simulink model "point_mass_subsonic_airplane"  (R2024b)
settings: Solver=ode45  StartTime=0.0  StopTime=5*60  RelTol=1e-6  AbsTol=1e-9
values from neighbouring files (symbols this model uses):
  FPS2MPH = 3600/5280    (= 0.681818181818)    [luckep2.m]
  RAD2DEG = 180/pi    (= 57.2957795131)    [luckep2.m]
undefined symbols (not defined in the file or in its folder): gd, ic, params
libraries: simulink_extras x5, dspstat3 x1, simulink x1
settings Model: Creator=jdlarson1  LastModifiedBy=Benjamin Lucke
settings SolverCC: AlgebraicLoopSolver=TrustRegion
settings DataIOCC: SaveFormat=Array  SignalLoggingSaveFormat=ModelDataLogs  ReturnWorkspaceOutputs=off
settings OptimizationCC: BlockReduction=off  BooleanDataType=off  ReuseModelBlockBuffer=off
settings DebuggingCC: SaveWithParameterizedLinksMsg=none  UnderspecifiedInitializationDetection=Classic  MergeDetectMultiDrivingBlocksExec=none  SignalResolutionControl=TryResolveAllWithWarning  MultiTaskDSMMsg=warning  MultiTaskCondExecSysMsg=none  UnconnectedInputMsg=warning  UnconnectedOutputMsg=warning  UnconnectedLineMsg=warning
settings HardwareCC: TargetUnknown=on
settings ModelReferenceCC: EnableRefExpFcnMdlSchedulingChecks=on  PropagateSignalLabelsOutOfModel=off
settings RTWCC: GPUComputeCapability=3.5  DLArmComputeVersion=19.05
settings GRTTargetCC: CombineOutputUpdateFcns=off  GRTInterface=on

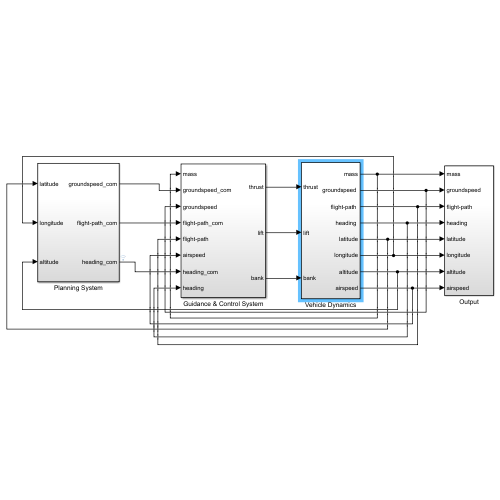
[thumbnail: Simulink's stored preview of the top-level diagram]
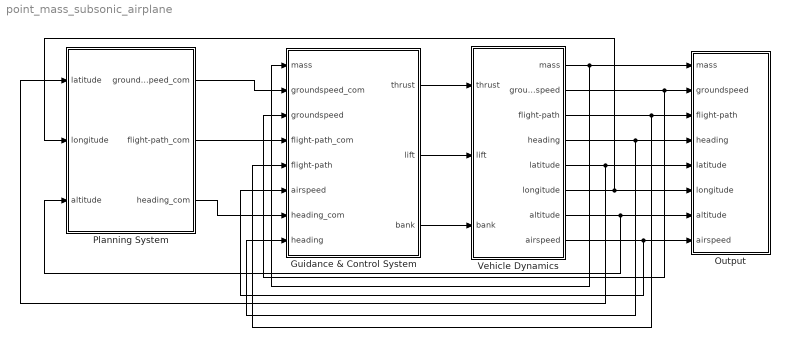
== system point_mass_subsonic_airplane ==
  Guidance & Control System : Subsystem
  Output : Subsystem
  Planning System : Subsystem
  Vehicle Dynamics : Subsystem
  wires:
  Guidance & Control System/3(bank) -> Vehicle Dynamics/3(bank)
  Vehicle Dynamics/1(" mass") -> Output/1(mass), Guidance & Control System/1(mass)
  Guidance & Control System/2(lift) -> Vehicle Dynamics/2("lift ")
  Guidance & Control System/1(thrust) -> Vehicle Dynamics/1("thrust ")
  Planning System/1(groundspeed_com) -> Guidance & Control System/2(groundspeed_com)
  Planning System/2(flight-path_com) -> Guidance & Control System/4(flight-path_com)
  Planning System/3(heading_com) -> Guidance & Control System/7(heading_com)
  Vehicle Dynamics/4(" heading ") -> Guidance & Control System/8(heading), Output/4(heading)
  Vehicle Dynamics/3(" flight-path ") -> Guidance & Control System/5(flight-path), Output/3(flight-path)
  Vehicle Dynamics/2(" groundspeed ") -> Guidance & Control System/3(groundspeed), Output/2(groundspeed)
  Vehicle Dynamics/8(airspeed) -> Guidance & Control System/6(airspeed), Output/8(airspeed)
  Vehicle Dynamics/7(altitude) -> Planning System/3(altitude), Output/7(altitude)
  Vehicle Dynamics/6(longitude) -> Planning System/2(longitude), Output/6(longitude)
  Vehicle Dynamics/5(latitude) -> Planning System/1(latitude), Output/5(latitude)

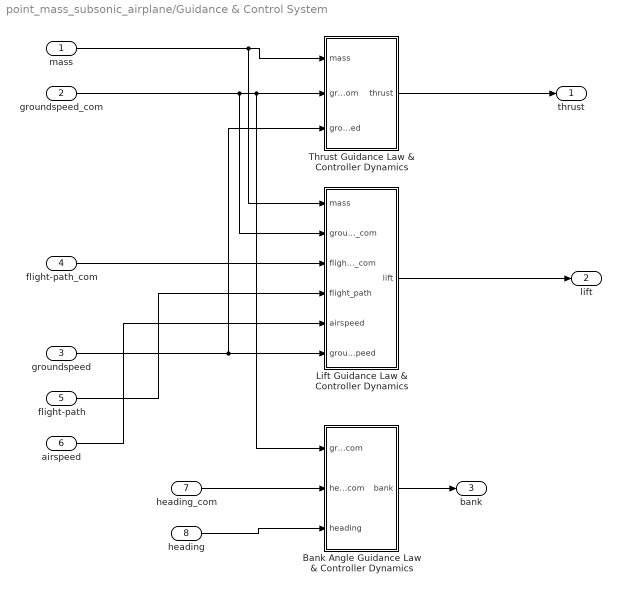
== system point_mass_subsonic_airplane/Guidance & Control System ==
  mass : Inport
  groundspeed_com : Inport  Port=2
  groundspeed : Inport  Port=3
  flight-path_com : Inport  Port=4
  flight-path : Inport  Port=5
  airspeed : Inport  Port=6
  heading_com : Inport  Port=7
  heading : Inport  Port=8
  Bank Angle Guidance Law & Controller Dynamics : Subsystem
  Lift Guidance Law & Controller Dynamics : Subsystem
  Thrust Guidance Law & Controller Dynamics : Subsystem
  thrust : Outport
  lift : Outport  Port=2
  bank : Outport  Port=3
  wires:
  mass/1 -> Lift Guidance Law & Controller Dynamics/1(mass), Thrust Guidance Law & Controller Dynamics/1(mass)
  flight-path_com/1 -> Lift Guidance Law & Controller Dynamics/3(flight_path_com)
  flight-path/1 -> Lift Guidance Law & Controller Dynamics/4(flight_path)
  groundspeed/1 -> Thrust Guidance Law & Controller Dynamics/3(groundspeed), Lift Guidance Law & Controller Dynamics/6(groundspeed)
  groundspeed_com/1 -> Bank Angle Guidance Law & Controller Dynamics/1(groundspeed_com), Thrust Guidance Law & Controller Dynamics/2(groundspeed_com), Lift Guidance Law & Controller Dynamics/2(groundspeed_com)
  heading/1 -> Bank Angle Guidance Law & Controller Dynamics/3(heading)
  airspeed/1 -> Lift Guidance Law & Controller Dynamics/5(airspeed)
  heading_com/1 -> Bank Angle Guidance Law & Controller Dynamics/2(heading_com)
  Thrust Guidance Law & Controller Dynamics/1(thrust) -> thrust/1
  Lift Guidance Law & Controller Dynamics/1(lift) -> lift/1
  Bank Angle Guidance Law & Controller Dynamics/1(bank) -> bank/1

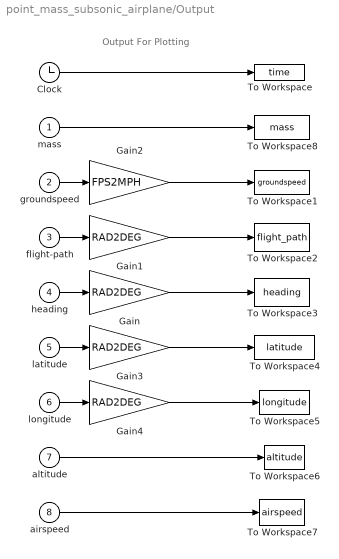
== system point_mass_subsonic_airplane/Output ==
  note: Output For Plotting
  mass : Inport
  groundspeed : Inport  Port=2
  flight-path : Inport  Port=3
  heading : Inport  Port=4
  latitude : Inport  Port=5
  longitude : Inport  Port=6
  altitude : Inport  Port=7
  airspeed : Inport  Port=8
  Clock : Clock
  Gain{,1,3..4} (4 alike) : Gain  Gain=RAD2DEG
  Gain2 : Gain  Gain=FPS2MPH
  To Workspace : ToWorkspace  VariableName=time
  To Workspace1 : ToWorkspace  VariableName=groundspeed
  To Workspace2 : ToWorkspace  VariableName=flight_path
  To Workspace3 : ToWorkspace  VariableName=heading
  To Workspace4 : ToWorkspace  VariableName=latitude
  To Workspace5 : ToWorkspace  VariableName=longitude
  To Workspace6 : ToWorkspace  VariableName=altitude
  To Workspace7 : ToWorkspace  VariableName=airspeed
  To Workspace8 : ToWorkspace  VariableName=mass
  wires:
  Clock/1 -> To Workspace/1
  latitude/1 -> Gain3/1
  groundspeed/1 -> Gain2/1
  flight-path/1 -> Gain1/1
  heading/1 -> Gain/1
  longitude/1 -> Gain4/1
  altitude/1 -> To Workspace6/1
  Gain2/1 -> To Workspace1/1
  Gain1/1 -> To Workspace2/1
  Gain/1 -> To Workspace3/1
  airspeed/1 -> To Workspace7/1
  mass/1 -> To Workspace8/1
  Gain3/1 -> To Workspace4/1
  Gain4/1 -> To Workspace5/1

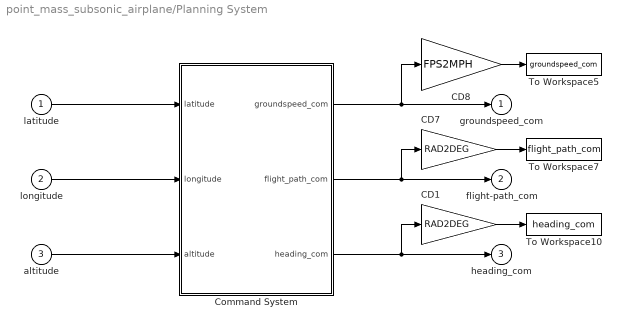
== system point_mass_subsonic_airplane/Planning System ==
  latitude : Inport
  longitude : Inport  Port=2
  altitude : Inport  Port=3
  CD1 : Gain  Gain=RAD2DEG  SaturateOnIntegerOverflow=on
  CD7 : Gain  Gain=RAD2DEG  SaturateOnIntegerOverflow=on
  CD8 : Gain  Gain=FPS2MPH  SaturateOnIntegerOverflow=on
  Command System : MATLAB Function  TreatAsAtomicUnit=on
  To Workspace10 : ToWorkspace  VariableName=heading_com
  To Workspace5 : ToWorkspace  VariableName=groundspeed_com
  To Workspace7 : ToWorkspace  VariableName=flight_path_com
  groundspeed_com : Outport
  flight-path_com : Outport  Port=2
  heading_com : Outport  Port=3
  wires:
  longitude/1 -> Command System/2(longitude)
  altitude/1 -> Command System/3(altitude)
  Command System/1(groundspeed_com) -> CD8/1, groundspeed_com/1
  Command System/2(flight_path_com) -> CD7/1, flight-path_com/1
  Command System/3(heading_com) -> CD1/1, heading_com/1
  CD8/1 -> To Workspace5/1
  CD7/1 -> To Workspace7/1
  CD1/1 -> To Workspace10/1
  latitude/1 -> Command System/1(latitude)

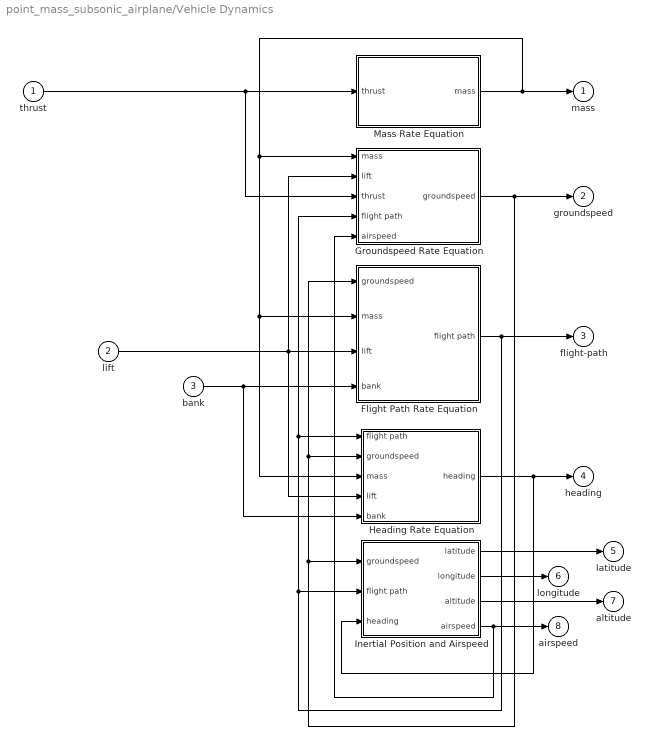
== system point_mass_subsonic_airplane/Vehicle Dynamics ==
  "thrust " : Inport
  "lift " : Inport  Port=2
  bank : Inport  Port=3
  Flight Path Rate Equation : Subsystem
  Groundspeed Rate Equation : Subsystem
  Heading Rate Equation : Subsystem
  Inertial Position and Airspeed : Subsystem
  Mass Rate Equation : Subsystem
  " mass" : Outport
  " groundspeed " : Outport  Port=2
  " flight-path " : Outport  Port=3
  " heading " : Outport  Port=4
  latitude : Outport  Port=5
  longitude : Outport  Port=6
  altitude : Outport  Port=7
  airspeed : Outport  Port=8
  wires:
  bank/1 -> Heading Rate Equation/5(bank), Flight Path Rate Equation/4(bank)
  "lift "/1 -> Heading Rate Equation/4("lift "), Flight Path Rate Equation/3("lift "), Groundspeed Rate Equation/2(lift)
  "thrust "/1 -> Groundspeed Rate Equation/3(thrust), Mass Rate Equation/1(thrust)
  Heading Rate Equation/1(heading) -> Inertial Position and Airspeed/3(heading), " heading "/1
  Flight Path Rate Equation/1(flight path) -> Groundspeed Rate Equation/4(flight path), Heading Rate Equation/1(flight path), Inertial Position and Airspeed/2("flight path "), " flight-path "/1
  Groundspeed Rate Equation/1(groundspeed) -> Flight Path Rate Equation/1(groundspeed), Heading Rate Equation/2(groundspeed), Inertial Position and Airspeed/1(groundspeed), " groundspeed "/1
  Inertial Position and Airspeed/2(longitude) -> longitude/1
  Inertial Position and Airspeed/4(airspeed) -> Groundspeed Rate Equation/5(airspeed), airspeed/1
  Inertial Position and Airspeed/1(latitude) -> latitude/1
  Inertial Position and Airspeed/3(altitude) -> altitude/1
  Mass Rate Equation/1("mass ") -> Heading Rate Equation/3(mass), Flight Path Rate Equation/2(mass), Groundspeed Rate Equation/1(mass), " mass"/1

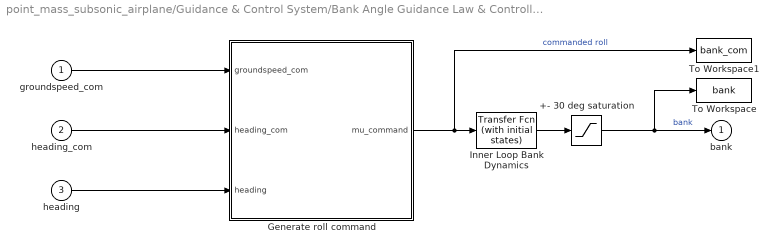
== system point_mass_subsonic_airplane/Guidance & Control System/Bank Angle Guidance Law & Controller Dynamics ==
  groundspeed_com : Inport
  heading_com : Inport  Port=2
  heading : Inport  Port=3
  +- 30 deg saturation : Saturate  UpperLimit=30*pi/180  LowerLimit=-30*pi/180
  Generate roll command : Subsystem
  Inner Loop Bank Dynamics : simulink_extras/Additional Linear/Transfer Fcn (with initial states)  N=[params.wu]  D="[1  params.wu]"  X0=0
  To Workspace : ToWorkspace  VariableName=bank
  To Workspace1 : ToWorkspace  VariableName=bank_com
  bank : Outport
  wires:
  groundspeed_com/1 -> Generate roll command/1(groundspeed_com)
  heading_com/1 -> Generate roll command/2(heading_com)
  heading/1 -> Generate roll command/3(heading)
  Generate roll command/1(mu_command) -> To Workspace1/1, Inner Loop Bank Dynamics/1  "commanded roll"
  Inner Loop Bank Dynamics/1 -> +- 30 deg saturation/1
  +- 30 deg saturation/1 -> bank/1, To Workspace/1  "bank"

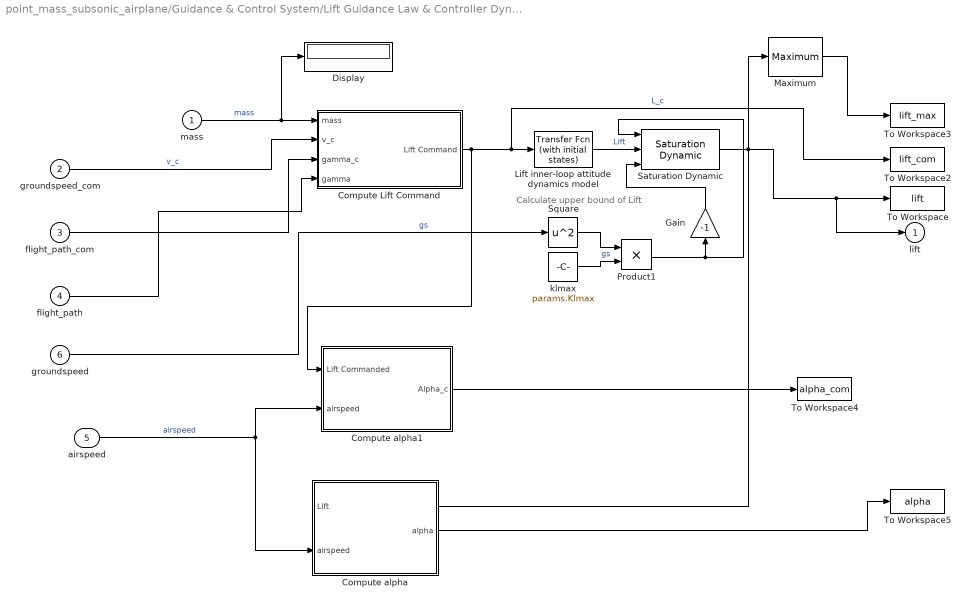
== system point_mass_subsonic_airplane/Guidance & Control System/Lift Guidance Law & Controller Dynamics ==
  note: Calculate upper bound of Lift
  mass : Inport
  groundspeed_com : Inport  Port=2
  flight_path_com : Inport  Port=3
  flight_path : Inport  Port=4
  airspeed : Inport  Port=5
  groundspeed : Inport  Port=6
  Compute Lift Command : Subsystem
  Compute alpha : Subsystem
  Compute alpha1 : Subsystem
  Display : Display
  Gain : Gain  Gain=-1
  Lift inner-loop attitude dynamics model : simulink_extras/Additional Linear/Transfer Fcn (with initial states)  N=[params.wl]  D="[1  params.wl]"  X0=0
  Maximum : dspstat3/Maximum  operation=maximum  fcn=Value  indexBase=One  operateOver=Each column  Dimension=1  InputProcessing=Columns as channels (frame based)  reset=None  roiEnable=off  roiType=Rectangles  roiPortion=Entire ROI  roiOutput=Individual statistics for each ROI  roiFlag=off  roundingMode=Floor  overflowMode=off  accumDataTypeStr=Inherit: Same as product output  accumLastDataTypeStr=Inherit: Same as product output
      settings: LibrarySourceBlock=dsphdlsupportstat/Maximum
  Product1 : Product
  Saturation Dynamic : simulink/Discontinuities/Saturation Dynamic  OutMin=[]  OutMax=[]  OutDataTypeStr=Inherit: Same as second input  OutDataType=fixdt(1, 16)  OutScaling=2^-10  DoSatur=off
  Square : Math  Operator=square
  To Workspace : ToWorkspace  VariableName=lift
  To Workspace2 : ToWorkspace  VariableName=lift_com
  To Workspace3 : ToWorkspace  VariableName=lift_max
  To Workspace4 : ToWorkspace  VariableName=alpha_com
  To Workspace5 : ToWorkspace  VariableName=alpha
  klmax : Constant  Value=params.Klmax
  lift : Outport
  wires:
  mass/1 -> Display/1, Compute Lift Command/1(mass)  "mass"
  groundspeed_com/1 -> Compute Lift Command/2(v_c)  "v_c"
  flight_path_com/1 -> Compute Lift Command/3(gamma_c)
  flight_path/1 -> Compute Lift Command/4(gamma)
  Compute Lift Command/1(Lift Command) -> Compute alpha1/1(Lift Commanded), To Workspace2/1, Lift inner-loop attitude dynamics model/1  "L_c"
  Lift inner-loop attitude dynamics model/1 -> Saturation Dynamic/2  "Lift"
  Maximum/1 -> To Workspace3/1
  groundspeed/1 -> Square/1  "gs"
  Square/1 -> Product1/1  "gs"
  klmax/1 -> Product1/2
  Product1/1 -> Gain/1, Saturation Dynamic/1
  Saturation Dynamic/1 -> Compute alpha/1(Lift), lift/1, To Workspace/1, Maximum/1
  airspeed/1 -> Compute alpha1/2(airspeed), Compute alpha/2(airspeed)  "airspeed"
  Compute alpha1/1(Alpha_c) -> To Workspace4/1
  Compute alpha/1(alpha) -> To Workspace5/1
  Gain/1 -> Saturation Dynamic/3

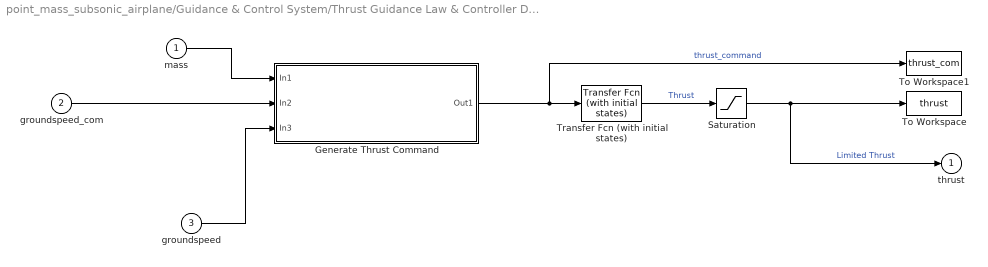
== system point_mass_subsonic_airplane/Guidance & Control System/Thrust Guidance Law & Controller Dynamics ==
  mass : Inport
  groundspeed_com : Inport  Port=2
  groundspeed : Inport  Port=3
  Generate Thrust Command : Subsystem
  Saturation : Saturate  UpperLimit=params.Tmax  LowerLimit=0
  To Workspace : ToWorkspace  VariableName=thrust
  To Workspace1 : ToWorkspace  VariableName=thrust_com
  Transfer Fcn (with initial states) : simulink_extras/Additional Linear/Transfer Fcn (with initial states)  N=[params.wt]  D="[1  params.wt]"  X0=22000
  thrust : Outport
  wires:
  mass/1 -> Generate Thrust Command/1(In1)
  groundspeed_com/1 -> Generate Thrust Command/2(In2)
  groundspeed/1 -> Generate Thrust Command/3(In3)
  Generate Thrust Command/1(Out1) -> Transfer Fcn (with initial states)/1, To Workspace1/1  "thrust_command"
  Transfer Fcn (with initial states)/1 -> Saturation/1  "Thrust"
  Saturation/1 -> thrust/1, To Workspace/1  "Limited Thrust"

== system point_mass_subsonic_airplane/Vehicle Dynamics/Flight Path Rate Equation ==
  groundspeed : Inport
  mass : Inport  Port=2
  "lift " : Inport  Port=3
  bank : Inport  Port=4
  Constant : Constant  Value=ic.g0
  Integrator : Integrator  InitialCondition=.05
  MATLAB Function : MATLAB Function  TreatAsAtomicUnit=on
  flight path : Outport
  wires:
  groundspeed/1 -> MATLAB Function/1(groundspeed)
  mass/1 -> MATLAB Function/2(mass)
  "lift "/1 -> MATLAB Function/3(lift)
  bank/1 -> MATLAB Function/4(bank)
  Constant/1 -> MATLAB Function/6(g0)
  MATLAB Function/1(flight_path_out) -> Integrator/1  "gamma_dot"
  Integrator/1 -> MATLAB Function/5(gamma), flight path/1

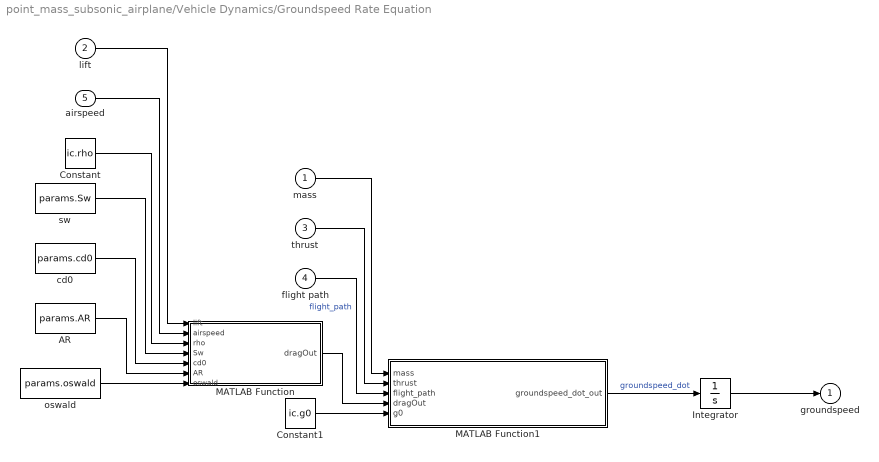
== system point_mass_subsonic_airplane/Vehicle Dynamics/Groundspeed Rate Equation ==
  mass : Inport
  lift : Inport  Port=2
  thrust : Inport  Port=3
  flight path : Inport  Port=4
  airspeed : Inport  Port=5
  AR : Constant  Value=params.AR
  Constant : Constant  Value=ic.rho
  Constant1 : Constant  Value=ic.g0
  Integrator : Integrator  InitialCondition=600
  MATLAB Function : MATLAB Function  TreatAsAtomicUnit=on
  MATLAB Function1 : MATLAB Function  TreatAsAtomicUnit=on
  cd0 : Constant  Value=params.cd0
  oswald : Constant  Value=params.oswald
  sw : Constant  Value=params.Sw
  groundspeed : Outport
  wires:
  mass/1 -> MATLAB Function1/1(mass)
  AR/1 -> MATLAB Function/6(AR)
  Constant/1 -> MATLAB Function/3(rho)
  airspeed/1 -> MATLAB Function/2(airspeed)
  lift/1 -> MATLAB Function/1(lift)
  oswald/1 -> MATLAB Function/7(oswald)
  cd0/1 -> MATLAB Function/5(cd0)
  sw/1 -> MATLAB Function/4(Sw)
  thrust/1 -> MATLAB Function1/2(thrust)
  flight path/1 -> MATLAB Function1/3(flight_path)  "flight_path"
  MATLAB Function/1(dragOut) -> MATLAB Function1/4(dragOut)
  Constant1/1 -> MATLAB Function1/5(g0)
  Integrator/1 -> groundspeed/1
  MATLAB Function1/1(groundspeed_dot_out) -> Integrator/1  "groundspeed_dot"

== system point_mass_subsonic_airplane/Vehicle Dynamics/Heading Rate Equation ==
  flight path : Inport
  groundspeed : Inport  Port=2
  mass : Inport  Port=3
  "lift " : Inport  Port=4
  bank : Inport  Port=5
  Integrator : Integrator
  MATLAB Function : MATLAB Function  TreatAsAtomicUnit=on
  heading : Outport
  wires:
  flight path/1 -> MATLAB Function/1(flight_path)
  groundspeed/1 -> MATLAB Function/2(groundspeed)
  mass/1 -> MATLAB Function/3(mass)
  "lift "/1 -> MATLAB Function/4(lift)
  bank/1 -> MATLAB Function/5(bank)
  MATLAB Function/1(heading_out) -> Integrator/1  "sigma-dot"
  Integrator/1 -> heading/1  "sigma"

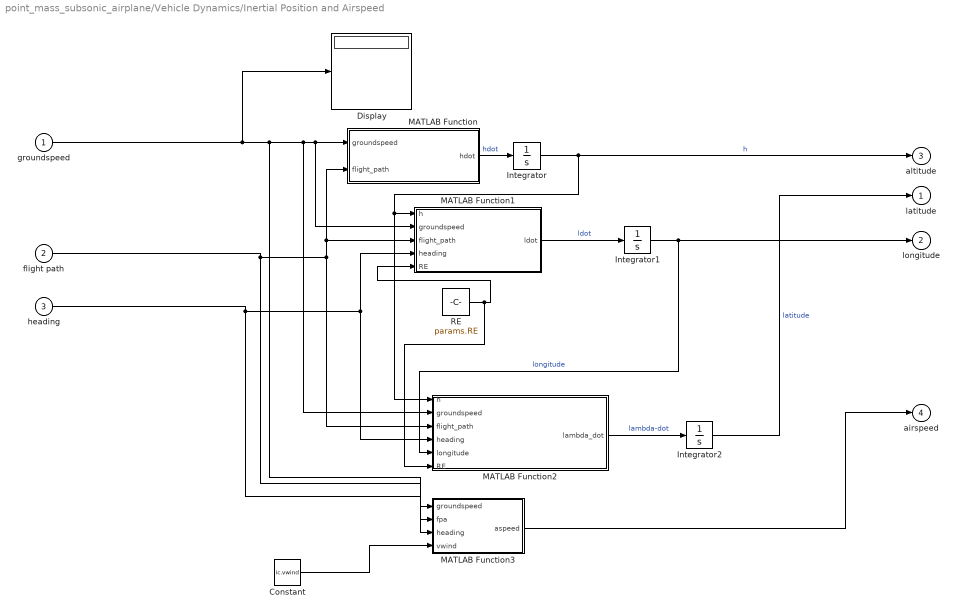
== system point_mass_subsonic_airplane/Vehicle Dynamics/Inertial Position and Airspeed ==
  groundspeed : Inport
  "flight path " : Inport  Port=2
  heading : Inport  Port=3
  Constant : Constant  Value=ic.vwind
  Display : Display
  Integrator : Integrator  InitialCondition=20000
  Integrator1 : Integrator  InitialCondition=33.2098
  Integrator2 : Integrator  InitialCondition=-87.5692
  MATLAB Function : MATLAB Function  TreatAsAtomicUnit=on
  MATLAB Function1 : MATLAB Function  TreatAsAtomicUnit=on
  MATLAB Function2 : MATLAB Function  TreatAsAtomicUnit=on
  MATLAB Function3 : MATLAB Function  TreatAsAtomicUnit=on
  RE : Constant  Value=params.RE
  latitude : Outport
  longitude : Outport  Port=2
  altitude : Outport  Port=3
  airspeed : Outport  Port=4
  wires:
  groundspeed/1 -> Display/1, MATLAB Function3/1(groundspeed), MATLAB Function2/2(groundspeed), MATLAB Function/1(groundspeed), MATLAB Function1/2(groundspeed)
  "flight path "/1 -> MATLAB Function2/3(flight_path), MATLAB Function/2(flight_path), MATLAB Function1/3(flight_path), MATLAB Function3/2(fpa)
  MATLAB Function/1(hdot) -> Integrator/1  "hdot"
  Integrator/1 -> MATLAB Function2/1(h), MATLAB Function1/1(h), altitude/1  "h"
  heading/1 -> MATLAB Function2/4(heading), MATLAB Function1/4(heading), MATLAB Function3/3(heading)
  MATLAB Function1/1(ldot) -> Integrator1/1  "ldot"
  Integrator1/1 -> MATLAB Function2/5(longitude), longitude/1  "longitude"
  MATLAB Function2/1(lambda_dot) -> Integrator2/1  "lambda-dot"
  Integrator2/1 -> latitude/1  "latitude"
  RE/1 -> MATLAB Function2/6(RE), MATLAB Function1/5(RE)
  Constant/1 -> MATLAB Function3/4(vwind)
  MATLAB Function3/1(aspeed) -> airspeed/1

== system point_mass_subsonic_airplane/Vehicle Dynamics/Mass Rate Equation ==
  thrust : Inport
  Gain : Gain  Gain=-1
  Integrator : Integrator  InitialCondition=200000
  K-f : Constant  Value=params.Kf
  Product : Product
  Product1 : Product
  To Workspace2 : ToWorkspace  VariableName=weight
  g : Constant  Value=ic.g0
  "mass " : Outport
  wires:
  thrust/1 -> Product/1
  K-f/1 -> Gain/1
  Product/1 -> Integrator/1  "mdot"
  Integrator/1 -> Product1/2, "mass "/1  "m"
  Gain/1 -> Product/2
  Product1/1 -> To Workspace2/1  "W"
  g/1 -> Product1/1  "g"

== system point_mass_subsonic_airplane/Guidance & Control System/Bank Angle Guidance Law & Controller Dynamics/Generate roll command ==
  groundspeed_com : Inport
  heading_com : Inport  Port=2
  heading : Inport  Port=3
  Divide : Product  Inputs=*/
  K_up : Gain  Gain=gd.Kup
  Mass1 : Constant  Value=ic.g0
  Product : Product
  Subtract : Sum  Inputs=+-
  mu_command : Outport
  wires:
  groundspeed_com/1 -> Divide/1
  Mass1/1 -> Divide/2
  Subtract/1 -> Product/2  "sigma_c - sigma"
  heading_com/1 -> Subtract/1
  heading/1 -> Subtract/2
  Divide/1 -> K_up/1
  K_up/1 -> Product/1
  Product/1 -> mu_command/1  "mu_command"

== system point_mass_subsonic_airplane/Guidance & Control System/Lift Guidance Law & Controller Dynamics/Compute Lift Command ==
  mass : Inport
  v_c : Inport  Port=2
  gamma_c : Inport  Port=3
  gamma : Inport  Port=4
  PI Thrust Controller : simulink_extras/Additional Linear/Transfer Fcn (with initial states)  N=[gd.Klp gd.Kli]  D="[1  0]"  X0=0
  Product : Product  Inputs=3
  compute sin difference : MATLAB Function  TreatAsAtomicUnit=on
  Lift Command : Outport
  wires:
  compute sin difference/1(y) -> Product/3
  Product/1 -> PI Thrust Controller/1
  gamma/1 -> compute sin difference/2(gamma)
  mass/1 -> Product/1
  v_c/1 -> Product/2
  gamma_c/1 -> compute sin difference/1(gamma_c)
  PI Thrust Controller/1 -> Lift Command/1  "Lift command"

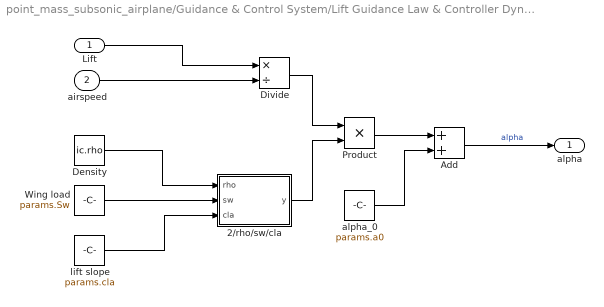
== system point_mass_subsonic_airplane/Guidance & Control System/Lift Guidance Law & Controller Dynamics/Compute alpha ==
  Lift : Inport
  airspeed : Inport  Port=2
  2/rho/sw/cla : MATLAB Function  TreatAsAtomicUnit=on
  Add : Sum
  Density : Constant  Value=ic.rho
  Divide : Product  Inputs=*/
  Product : Product
  Wing load : Constant  Value=params.Sw
  alpha_0 : Constant  Value=params.a0
  lift slope : Constant  Value=params.cla
  alpha : Outport
  wires:
  Add/1 -> alpha/1  "alpha"
  2/rho/sw/cla/1(y) -> Product/2
  Density/1 -> 2/rho/sw/cla/1(rho)
  airspeed/1 -> Divide/2
  Lift/1 -> Divide/1
  Divide/1 -> Product/1
  lift slope/1 -> 2/rho/sw/cla/3(cla)
  Wing load/1 -> 2/rho/sw/cla/2(sw)
  Product/1 -> Add/1
  alpha_0/1 -> Add/2

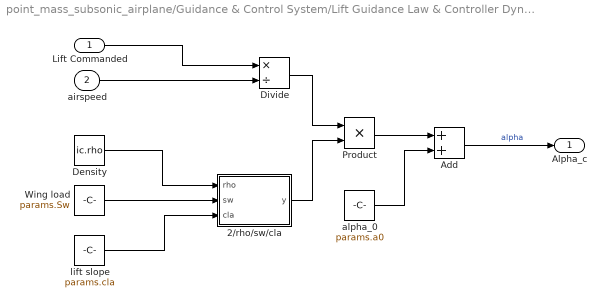
== system point_mass_subsonic_airplane/Guidance & Control System/Lift Guidance Law & Controller Dynamics/Compute alpha1 ==
  Lift Commanded : Inport
  airspeed : Inport  Port=2
  2/rho/sw/cla : MATLAB Function  TreatAsAtomicUnit=on
  Add : Sum
  Density : Constant  Value=ic.rho
  Divide : Product  Inputs=*/
  Product : Product
  Wing load : Constant  Value=params.Sw
  alpha_0 : Constant  Value=params.a0
  lift slope : Constant  Value=params.cla
  Alpha_c : Outport
  wires:
  alpha_0/1 -> Add/2
  Product/1 -> Add/1
  Wing load/1 -> 2/rho/sw/cla/2(sw)
  lift slope/1 -> 2/rho/sw/cla/3(cla)
  Divide/1 -> Product/1
  Lift Commanded/1 -> Divide/1
  airspeed/1 -> Divide/2
  Density/1 -> 2/rho/sw/cla/1(rho)
  2/rho/sw/cla/1(y) -> Product/2
  Add/1 -> Alpha_c/1  "alpha"

== system point_mass_subsonic_airplane/Guidance & Control System/Thrust Guidance Law & Controller Dynamics/Generate Thrust Command ==
  In1 : Inport
  In2 : Inport  Port=2
  In3 : Inport  Port=3
  Add : Sum  Inputs=+-
  PI Thrust Controller : simulink_extras/Additional Linear/Transfer Fcn (with initial states)  N=[gd.Ktp gd.Kti]  D="[1  0]"  X0=0
  Product : Product
  Out1 : Outport
  wires:
  Product/1 -> PI Thrust Controller/1
  Add/1 -> Product/2
  PI Thrust Controller/1 -> Out1/1  "Thrust command"
  In3/1 -> Add/2  "Groundspeed actual"
  In1/1 -> Product/1  "Mass"
  In2/1 -> Add/1  "Groundspeed Command"

== matlab function point_mass_subsonic_airplane/Vehicle Dynamics/Groundspeed Rate Equation/MATLAB Function1 ==
  data: mass input; groundspeed_dot_out output; thrust input; flight_path input; dragOut input; g0 input
function groundspeed_dot_out = fcn(mass, thrust, flight_path, dragOut, g0)
groundspeed_dot_out = (thrust - dragOut)/mass - g0*sind(flight_path);

== matlab function point_mass_subsonic_airplane/Guidance & Control System/Lift Guidance Law & Controller Dynamics/Compute Lift Command/compute sin difference ==
  data: gamma_c input; y output; gamma input
function y = sindifference_fpa(gamma_c, gamma)
y = sind(gamma_c) - sind(gamma);

== matlab function point_mass_subsonic_airplane/Guidance & Control System/Lift Guidance Law & Controller Dynamics/Compute alpha1/2//rho//sw//cla ==
  data: y output; rho input; sw input; cla input
function y = fcn(rho, sw, cla)
y = 2/(rho*sw*cla);

== matlab function point_mass_subsonic_airplane/Guidance & Control System/Lift Guidance Law & Controller Dynamics/Compute alpha/2//rho//sw//cla ==
  data: y output; rho input; sw input; cla input
function y = fcn(rho, sw, cla)
y = 2/(rho*sw*cla);

== matlab function point_mass_subsonic_airplane/Planning System/Command System ==
  data: latitude input; groundspeed_com output; longitude input; altitude input; flight_path_com output; heading_com output
function [groundspeed_com, flight_path_com, heading_com] = ...
    command_trajectory(latitude, longitude, altitude)
% Define the commanded velocity, flight path and heading

FPS2MPH = 3600/5280;
DEG2RAD = pi/180;
RAD2DEG = 180/pi;

groundspeed_com = 450/FPS2MPH;          % fps
flight_path_com = 5*DEG2RAD;    % rad
heading_com = 15*DEG2RAD;          % rad

end

== matlab function point_mass_subsonic_airplane/Vehicle Dynamics/Groundspeed Rate Equation/MATLAB Function ==
  data: lift input; dragOut output; airspeed input; rho input; Sw input; cd0 input; AR input; oswald input
function dragOut = getDrag(lift, airspeed, rho, Sw, cd0, AR, oswald)
t1 = 1/2 * rho * Sw * cd0 * airspeed;
t2 = 2/(rho * Sw * pi * AR * oswald);
t3 = lift^2/airspeed;
dragOut = t1 + t2*t3;

== matlab function point_mass_subsonic_airplane/Vehicle Dynamics/Flight Path Rate Equation/MATLAB Function ==
  data: groundspeed input; flight_path_out output; mass input; lift input; bank input; gamma input; g0 input
function flight_path_out = fcn(groundspeed, mass, lift,  bank, gamma, g0)
flight_path_out = 1/groundspeed * (lift/mass*cosd(bank) - ...
    g0 * cosd(gamma));

== matlab function point_mass_subsonic_airplane/Vehicle Dynamics/Heading Rate Equation/MATLAB Function ==
  data: flight_path input; heading_out output; groundspeed input; mass input; lift input; bank input
function heading_out = getHeading(flight_path, groundspeed, mass, lift,  bank)
heading_out = 1/(groundspeed*cosd(flight_path)) * (lift/mass*sind(bank));

== matlab function point_mass_subsonic_airplane/Vehicle Dynamics/Inertial Position and Airspeed/MATLAB Function ==
  data: groundspeed input; hdot output; flight_path input
function hdot = calchdot(groundspeed, flight_path)
hdot = groundspeed * sind(flight_path);

== matlab function point_mass_subsonic_airplane/Vehicle Dynamics/Inertial Position and Airspeed/MATLAB Function1 ==
  data: h input; groundspeed input; ldot output; flight_path input; heading input; RE input
function ldot = calc_ldot(h, groundspeed, flight_path, heading, RE)
ldot = groundspeed * cosd(flight_path)*cosd(heading)/(RE + h);

== matlab function point_mass_subsonic_airplane/Vehicle Dynamics/Inertial Position and Airspeed/MATLAB Function2 ==
  data: h input; lambda_dot output; groundspeed input; flight_path input; heading input; longitude input; RE input
function lambda_dot = calcLambdaDot(h, groundspeed, flight_path, heading, longitude, RE)
lambda_dot = groundspeed * cosd(flight_path) * sind(heading)/...
    ((RE + h)*cosd(longitude));

== matlab function point_mass_subsonic_airplane/Vehicle Dynamics/Inertial Position and Airspeed/MATLAB Function3 ==
  data: groundspeed input; aspeed output; fpa input; heading input; vwind input
function aspeed = getAirspeed(groundspeed, fpa, heading, vwind)
uvw = [groundspeed*cosd(fpa)*cosd(heading)
    groundspeed*cosd(fpa)*sind(heading)
    groundspeed*sind(fpa)];
vinf = uvw - [40 40 0]';
aspeed = vinf(1).^2 + vinf(2).^2 + vinf(3).^2;
